simulink subsystem "EoMM"  (R2021b)
settings: Solver=VariableStepAuto  StartTime=0.0  StopTime=10.0  RelTol=1e-3
values from neighbouring files (symbols this model uses):
  g = 9.80665    [codigos.m]    (also in eom.m)
  Ix = 0.83    [codigos.m]    (also in eom.m)
  Ixz = 0.13    [codigos.m]    (also in eom.m)
  Iy = 1.2    [codigos.m]    (also in eom.m)
  Iz = 1.8    [codigos.m]    (also in eom.m)
  m = 15    [codigos.m]    (also in eom.m)
settings Model: Creator=verti  LastModifiedBy=verti

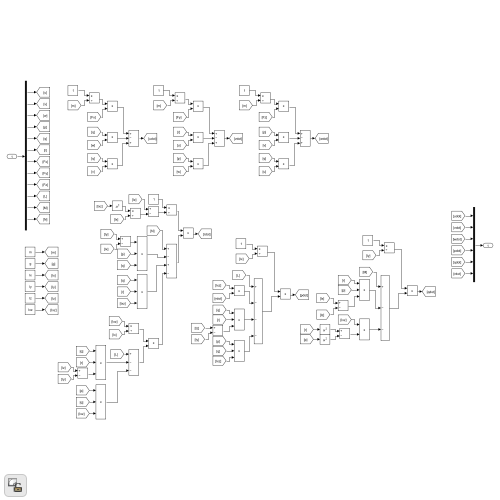
[thumbnail: Simulink's stored preview of the top-level diagram]
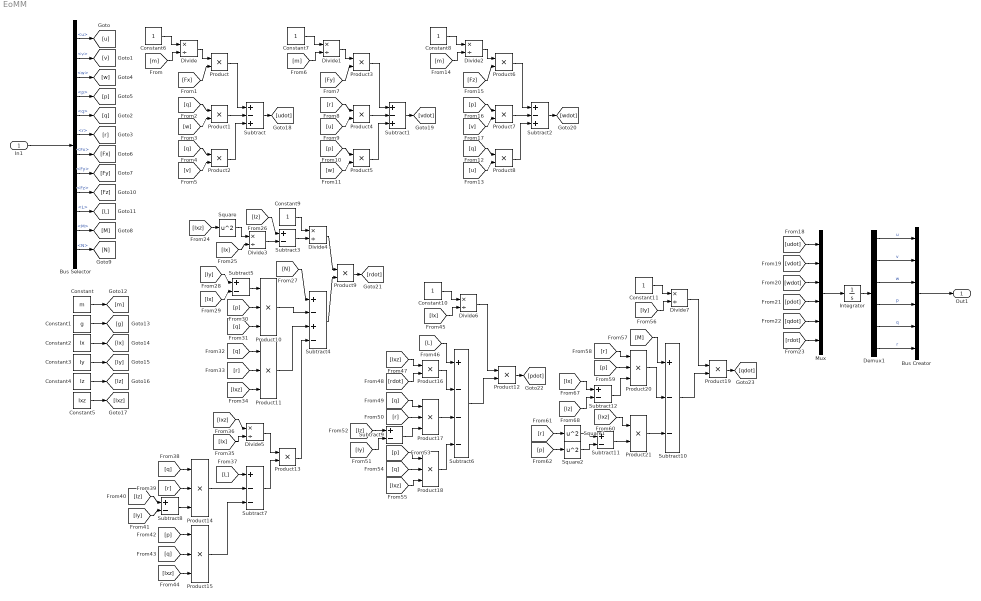
== system EoMM ==
  In1 : Inport
  Bus Creator : BusCreator  Inputs=6
  Bus Selector : BusSelector  OutputSignals=velocidades.u,velocidades.v,velocidades.w,velocidades.p,velocidades.q,velocidades.r,fuerzas.Fx,fuerzas.Fy,fuerzas.Fz,fuerzas.L,fuerzas.M,fuerzas.N
  Constant : Constant  Value=m
  Constant1 : Constant  Value=g
  Constant{6..11} (6 alike) : Constant
  Constant2 : Constant  Value=Ix
  Constant3 : Constant  Value=Iy
  Constant4 : Constant  Value=Iz
  Constant5 : Constant  Value=Ixz
  Demux1 : Demux  Outputs=6
  Divide{,1..7} (8 alike) : Product  Inputs=*/
  Integrator : Integrator  InitialCondition=[0.001,0,0,0,0,0]
  Mux : Mux  Inputs=6
  Product{,1..9,12..13,16,19,21} (15 alike) : Product
  Product{10..11,14..15,17..18,20} (7 alike) : Product  Inputs=3
  Square : Math  Operator=square  SaturateOnIntegerOverflow=on
  Square1 : Math  Operator=square  SaturateOnIntegerOverflow=on
  Square2 : Math  Operator=square  SaturateOnIntegerOverflow=on
  Subtract : Sum  Inputs=+-+
  Subtract1 : Sum  Inputs=+-+
  Subtract10 : Sum  Inputs=+--
  Subtract{3,5,8..9,11..12} (6 alike) : Sum  Inputs=+-
  Subtract2 : Sum  Inputs=+-+
  Subtract4 : Sum  Inputs=+-+-
  Subtract6 : Sum  Inputs=+---
  Subtract7 : Sum  Inputs=+--
  Out1 : Outport
  wires:
  In1/1 -> Bus Selector/1
  Bus Selector/3 -> [w]  "<w>"
  Bus Selector/1 -> [u]  "<u>"
  Bus Selector/2 -> [v]  "<v>"
  Bus Selector/4 -> [p]  "<p>"
  Bus Selector/5 -> [q]  "<q>"
  Bus Selector/6 -> [r]  "<r>"
  Bus Selector/7 -> [Fx]  "<Fx>"
  Bus Selector/12 -> [N]  "<N>"
  Bus Selector/11 -> [M]  "<M>"
  Bus Selector/10 -> [L]  "<L>"
  Bus Selector/9 -> [Fz]  "<Fz>"
  Bus Selector/8 -> [Fy]  "<Fy>"
  Constant/1 -> [m]
  Constant1/1 -> [g]
  Constant3/1 -> [Iy]
  Constant2/1 -> [Ix]
  Constant5/1 -> [Ixz]
  Constant4/1 -> [Iz]
  Constant6/1 -> Divide/1
  [m] -> Divide/2
  [Fx] -> Product/2
  Divide/1 -> Product/1
  [q] -> Product1/1
  [w] -> Product1/2
  [q] -> Product2/1
  [v] -> Product2/2
  Product2/1 -> Subtract/3
  Product/1 -> Subtract/1
  Product1/1 -> Subtract/2
  Subtract/1 -> [udot]
  Subtract1/1 -> [vdot]
  Product4/1 -> Subtract1/2
  Product3/1 -> Subtract1/1
  Product5/1 -> Subtract1/3
  [w] -> Product5/2
  [p] -> Product5/1
  [u] -> Product4/2
  [r] -> Product4/1
  Divide1/1 -> Product3/1
  [Fy] -> Product3/2
  [m] -> Divide1/2
  Constant7/1 -> Divide1/1
  Constant8/1 -> Divide2/1
  [m] -> Divide2/2
  [Fz] -> Product6/2
  Divide2/1 -> Product6/1
  [p] -> Product7/1
  [v] -> Product7/2
  [q] -> Product8/1
  [u] -> Product8/2
  Product8/1 -> Subtract2/3
  Product6/1 -> Subtract2/1
  Product7/1 -> Subtract2/2
  Subtract2/1 -> [wdot]
  [rdot] -> Mux/6
  [udot] -> Mux/1
  [vdot] -> Mux/2
  [wdot] -> Mux/3
  [pdot] -> Mux/4
  [qdot] -> Mux/5
  [Ixz] -> Square/1
  Square/1 -> Divide3/1
  [Ix] -> Divide3/2
  [Iz] -> Subtract3/1
  Divide3/1 -> Subtract3/2
  Subtract3/1 -> Divide4/2
  Constant9/1 -> Divide4/1
  Divide4/1 -> Product9/1
  Subtract4/1 -> Product9/2
  [N] -> Subtract4/1
  [Iy] -> Subtract5/1
  [Ix] -> Subtract5/2
  Subtract5/1 -> Product10/1
  Product10/1 -> Subtract4/2
  [p] -> Product10/2
  [q] -> Product10/3
  [Ixz] -> Product11/3
  [r] -> Product11/2
  Product11/1 -> Subtract4/3
  [q] -> Product11/1
  [Ix] -> Divide5/2
  [Ixz] -> Divide5/1
  Product13/1 -> Subtract4/4
  Divide5/1 -> Product13/1
  Subtract7/1 -> Product13/2
  [L] -> Subtract7/1
  Product14/1 -> Subtract7/2
  Subtract8/1 -> Product14/3
  [q] -> Product14/1
  [r] -> Product14/2
  [Iz] -> Subtract8/1
  [Iy] -> Subtract8/2
  [q] -> Product15/2
  [p] -> Product15/1
  Product15/1 -> Subtract7/3
  [Ixz] -> Product15/3
  Product9/1 -> [rdot]
  Product12/1 -> [pdot]
  [Ix] -> Divide6/2
  Constant10/1 -> Divide6/1
  Divide6/1 -> Product12/1
  Subtract6/1 -> Product12/2
  [L] -> Subtract6/1
  [Ixz] -> Product16/1
  [rdot] -> Product16/2
  Product16/1 -> Subtract6/2
  Product17/1 -> Subtract6/3
  [q] -> Product17/1
  [r] -> Product17/2
  Subtract9/1 -> Product17/3
  [Iz] -> Subtract9/1
  [Iy] -> Subtract9/2
  [q] -> Product18/2
  [p] -> Product18/1
  [Ixz] -> Product18/3
  Product18/1 -> Subtract6/4
  [Ixz] -> Product21/1
  Product21/1 -> Subtract10/3
  Product20/1 -> Subtract10/2
  [M] -> Subtract10/1
  Subtract10/1 -> Product19/2
  Divide7/1 -> Product19/1
  Constant11/1 -> Divide7/1
  [Iy] -> Divide7/2
  Product19/1 -> [qdot]
  [r] -> Product20/1
  [p] -> Product20/2
  Subtract12/1 -> Product20/3
  [Ix] -> Subtract12/1
  [Iz] -> Subtract12/2
  Subtract11/1 -> Product21/2
  [r] -> Square1/1
  [p] -> Square2/1
  Square2/1 -> Subtract11/2
  Square1/1 -> Subtract11/1
  Mux/1 -> Integrator/1
  Integrator/1 -> Demux1/1
  Demux1/6 -> Bus Creator/6  "r"
  Demux1/5 -> Bus Creator/5  "q"
  Demux1/4 -> Bus Creator/4  "p"
  Demux1/3 -> Bus Creator/3  "w"
  Demux1/2 -> Bus Creator/2  "v"
  Demux1/1 -> Bus Creator/1  "u"
  Bus Creator/1 -> Out1/1
